simulink model "Simulate_it3"  (R2014a)
settings: Solver=ode1  StartTime=0.0  StopTime=inf  FixedStep=0.002  RelTol=1e-3
StartFcn:
  | callBack
values from neighbouring files (symbols this model uses):
  ki = -( -AmpMax + kp * e_ss ) / ti / e_ss    [d_i_design.m]    (also in setup_srv02_exp02_pos.m = 0)
  kp = wn^2/K*tau    [d_pv_design.m]    (also in setup_srv02_exp02_pos.m = 0)
  kv = (-1+2*zeta*wn*tau)/K    [d_pv_design.m]    (also in setup_srv02_exp02_pos.m = 0)
  VMAX_DAC = 10    [setup_srv02_exp02_pos.m]
  wcf = 2 * pi * 50.0    (= 314.159265359)    [setup_srv02_exp02_pos.m]
  zetaf = 0.9    [setup_srv02_exp02_pos.m]
undefined symbols (not defined in the file or in its folder): K_POT, K_TACH, Q2, USB, VMAX_AMP
libraries: quarc_library x3
settings Model: SimulationMode=external  ExtModeTrigDuration=5000  Creator=msr5h7  LastModifiedBy=mmgxw3
settings SolverCC: PositivePriorityOrder=on
settings RTWCC: SystemTargetFile=quarc_win64.tlc  TemplateMakefile=quarc_default_tmf  Description=QUARC Win64 Target  ProcessScript=quarc_win64_make_rtw_hook
settings STFCustomTargetCC: CombineOutputUpdateFcns=on  GRTInterface=off
settings GRTTargetCC: ParMdlRefBuildCompliant=off  CompOptLevelCompliant=off  MatFileLogging=off  CPPClassGenCompliant=off  ExtMode=on  ExtModeMexFile=quarc_comm

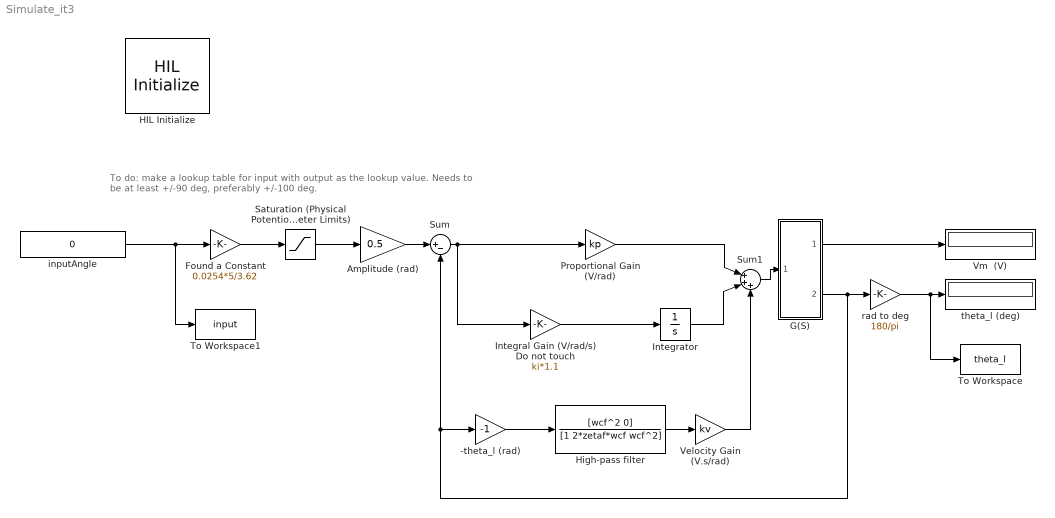
== system Simulate_it3 ==
  note: To do: make a lookup table for input with output as the lookup value.
      | Needs to be at least +/-90 deg, preferably +/-100 deg.
  -theta_l (rad) : Gain  Gain=-1
  Amplitude (rad) : Gain  Gain=0.5  SaturateOnIntegerOverflow=on  OutDataTypeStr=Inherit: Same as input  ParamDataTypeStr=Inherit: Same as input
  Found a Constant : Gain  Gain=0.0254*5/3.62
  G(S) : Subsystem
  HIL Initialize : quarc_library/Data Acquisition/Generic/Configuration/HIL Initialize  Priority=-99  object_name=Q2-USB  board_type=q2_usb  board_number=0  board_options=d0=digital;d1=digital;led=auto;update_rate=normal;decimation=1  exclusive=off  active=off  hardware_clocks=[0]  clock_modes=[]  initial_clock_frequencies=[]  set_clock_params_at_start=off  set_clock_params_at_switch_in=off  set_clock_frequencies_at_start=off  set_clock_frequencies_at_switch_in=off  analog_input_channels=[0:1]  analog_input_maximums=10  analog_input_minimums=-10  set_analog_input_params_at_start=on  set_analog_input_params_at_switch_in=off  analog_output_channels=[0]  analog_output_maximums=10  analog_output_minimums=-10  initial_analog_outputs=[0]  final_analog_outputs=[0]  watchdog_analog_outputs=0  set_analog_output_params_at_start=on  set_analog_output_params_at_switch_in=off  set_analog_outputs_at_start=on  set_analog_outputs_at_switch_in=off  set_analog_outputs_at_terminate=on  set_analog_outputs_at_switch_out=off  set_analog_outputs_on_watchdog=off  digital_input_channels=[]  digital_output_channels=[]  digital_output_configuration=[]  initial_digital_outputs=[1]  final_digital_outputs=[1]  watchdog_digital_outputs=[1]  set_digital_output_params_at_start=off  set_digital_output_params_at_switch_in=off  set_digital_outputs_at_start=off  set_digital_outputs_at_switch_in=off  set_digital_outputs_at_terminate=off  set_digital_outputs_at_switch_out=off  set_digital_outputs_on_watchdog=off  encoder_channels=[]  quadrature=[4]  encoder_filter_frequency=[]  initial_encoder_counts=[0]  set_encoder_params_at_start=on  set_encoder_params_at_switch_in=off  set_encoder_counts_at_start=on  set_encoder_counts_at_switch_in=off  pwm_channels=[]  pwm_modes=[0]  pwm_frequency=1/0.020  pwm_configuration=[]  pwm_alignment=[]  pwm_polarity=[]  pwm_leading_deadband=[]  pwm_trailing_deadband=[]  initial_pwm_outputs=[0]  final_pwm_outputs=[0]  watchdog_pwm_outputs=[0]  set_pwm_params_at_start=on  set_pwm_params_at_switch_in=off  set_pwm_outputs_at_start=on  set_pwm_outputs_at_switch_in=off  set_pwm_outputs_at_terminate=on  set_pwm_outputs_at_switch_out=off  set_pwm_outputs_on_watchdog=off  other_output_channels=[]  initial_other_outputs=[]  final_other_outputs=[]  watchdog_other_outputs=[]  set_other_outputs_at_start=off  set_other_outputs_at_switch_in=off  set_other_outputs_at_terminate=off  set_other_outputs_at_switch_out=off  set_other_outputs_on_watchdog=off
  High-pass filter : TransferFcn  Numerator=[wcf^2 0]  Denominator=[1 2*zetaf*wcf wcf^2]
  Integral Gain (V/rad/s) Do not touch : Gain  Gain=ki*1.1
  Integrator : Integrator  LimitOutput=on  UpperSaturationLimit=VMAX_DAC  LowerSaturationLimit=-VMAX_DAC
  Proportional Gain (V/rad) : Gain  Gain=kp
  Saturation (Physical Potentiometer Limits) : Saturate  UpperLimit=7.55  LowerLimit=-7.65
  Sum : Sum  Inputs=|+-
  Sum1 : Sum  Inputs=|+++
  To Workspace : ToWorkspace  VariableName=theta_l  SampleTime=-1
  To Workspace1 : ToWorkspace  VariableName=input  SampleTime=-1
  Velocity Gain (V.s/rad) : Gain  Gain=kv
  Vm  (V) : Display
  inputAngle : Constant  Value=0
  rad to deg : Gain  Gain=180/pi
  theta_l (deg) : Display
  wires:
  G(S)/1(Out1) -> Vm  (V)/1
  G(S)/2(Out2) -> Sum/2, -theta_l (rad)/1, rad to deg/1
  Amplitude (rad)/1 -> Sum/1
  Sum/1 -> Proportional Gain (V/rad)/1, Integral Gain (V/rad/s) Do not touch/1
  Sum1/1 -> G(S)/1(In1)
  Proportional Gain (V/rad)/1 -> Sum1/1
  Integral Gain (V/rad/s) Do not touch/1 -> Integrator/1
  Integrator/1 -> Sum1/2
  -theta_l (rad)/1 -> High-pass filter/1
  High-pass filter/1 -> Velocity Gain (V.s/rad)/1
  Velocity Gain (V.s/rad)/1 -> Sum1/3
  Found a Constant/1 -> Saturation (Physical Potentiometer Limits)/1
  Saturation (Physical Potentiometer Limits)/1 -> Amplitude (rad)/1
  rad to deg/1 -> To Workspace/1, theta_l (deg)/1
  inputAngle/1 -> Found a Constant/1, To Workspace1/1

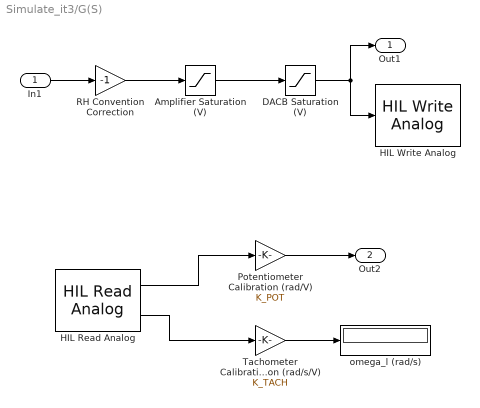
== system Simulate_it3/G(S) ==
  In1 : Inport
  Amplifier Saturation (V) : Saturate  UpperLimit=VMAX_AMP  LowerLimit=-VMAX_AMP
  DACB Saturation (V) : Saturate  UpperLimit=.5  LowerLimit=-.5
  HIL Read Analog : quarc_library/Data Acquisition/Generic/Immediate I//O/HIL Read Analog  object_name=Q2-USB  channels=[0:1]  sample_time=qc_get_step_size  active=on  vector_output=off
  HIL Write Analog : quarc_library/Data Acquisition/Generic/Immediate I//O/HIL Write Analog  object_name=Q2-USB  channels=0  sample_time=-1  active=off  vector_input=off
  Potentiometer Calibration (rad/V) : Gain  Gain=K_POT
  RH Convention Correction : Gain  Gain=-1
  Tachometer Calibration (rad/s/V) : Gain  Gain=K_TACH
  omega_l (rad/s) : Display
  Out1 : Outport
  Out2 : Outport  Port=2
  wires:
  Amplifier Saturation (V)/1 -> DACB Saturation (V)/1
  In1/1 -> RH Convention Correction/1
  Tachometer Calibration (rad/s/V)/1 -> omega_l (rad/s)/1
  RH Convention Correction/1 -> Amplifier Saturation (V)/1
  HIL Read Analog/1 -> Potentiometer Calibration (rad/V)/1
  Potentiometer Calibration (rad/V)/1 -> Out2/1
  HIL Read Analog/2 -> Tachometer Calibration (rad/s/V)/1
  DACB Saturation (V)/1 -> Out1/1, HIL Write Analog/1
